simulink model "Interpolator"  (R2019a)
settings: Solver=FixedStepAuto  StartTime=0.0  StopTime=inf  FixedStep=0.001  RelTol=1e-3
settings Model: NumberOfSteps=1000  Creator=EiLit  LastModifiedBy=EiLit
settings DataIOCC: ReturnWorkspaceOutputs=off
settings DebuggingCC: ArithmeticOperatorsInVariantConditions=warning

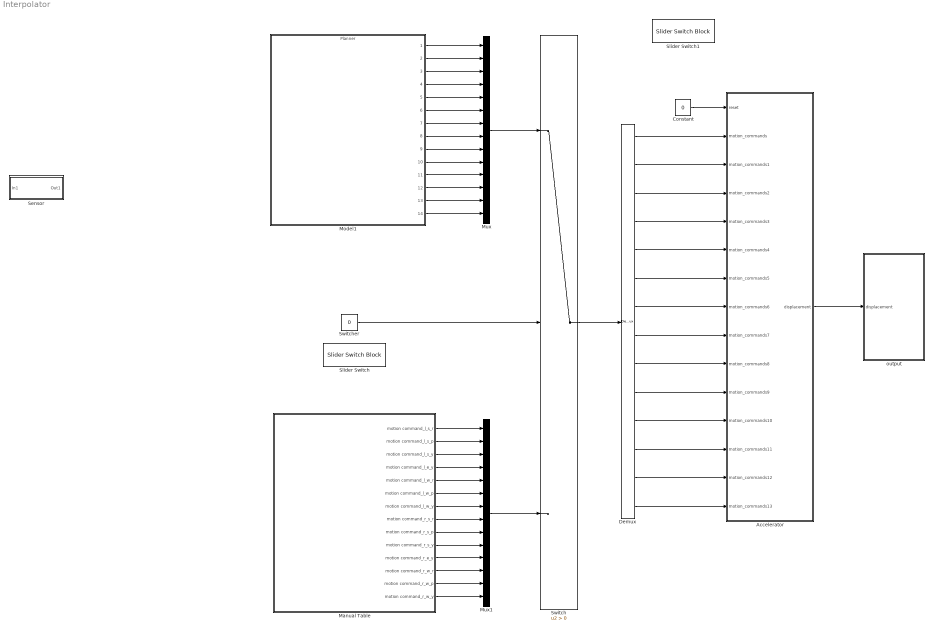
== system Interpolator ==
  Accelerator : Subsystem
  Constant : Constant  Value=0
  Demux : Demux  Outputs=14
  Manual Table : Subsystem
  Model1 : ModelReference  ModelNameDialog=Planner  SimulationMode=Normal  ModelReferenceVersion=1.6
  Mux : Mux  Inputs=14
  Mux1 : Mux  Inputs=14
  Sensor : Subsystem
  Slider Switch : SliderSwitchBlock
      settings: Values={{'Auto', 'Mannual'}, [1 0]}
  Slider Switch1 : SliderSwitchBlock
      settings: Values={{'off', 'reset'}, [0 1]}
  Switch : Switch  Criteria=u2 > Threshold
  Switcher : Constant  Value=0
  output : Subsystem
  wires:
  Accelerator/1(displacement) -> output/1(displacement)
  Switch/1 -> Demux/1
  Switcher/1 -> Switch/2
  Model1/1 -> Mux/1
  Model1/2 -> Mux/2
  Model1/3 -> Mux/3
  Model1/4 -> Mux/4
  Model1/5 -> Mux/5
  Model1/6 -> Mux/6
  Model1/7 -> Mux/7
  Model1/8 -> Mux/8
  Model1/9 -> Mux/9
  Model1/10 -> Mux/10
  Model1/11 -> Mux/11
  Model1/12 -> Mux/12
  Model1/13 -> Mux/13
  Model1/14 -> Mux/14
  Mux/1 -> Switch/1
  Mux1/1 -> Switch/3
  Manual Table/1(motion command_l_s_r) -> Mux1/1
  Manual Table/2(motion command_l_s_p) -> Mux1/2
  Manual Table/3(motion command_l_s_y) -> Mux1/3
  Manual Table/4(motion command_l_e_y) -> Mux1/4
  Manual Table/5(motion command_l_w_r) -> Mux1/5
  Manual Table/6(motion command_l_w_p) -> Mux1/6
  Manual Table/7(motion command_l_w_y) -> Mux1/7
  Manual Table/8(motion command_r_s_r) -> Mux1/8
  Manual Table/9(motion command_r_s_p) -> Mux1/9
  Manual Table/10(motion command_r_s_y) -> Mux1/10
  Manual Table/11(motion command_r_e_y) -> Mux1/11
  Manual Table/12(motion command_r_w_r) -> Mux1/12
  Manual Table/13(motion command_r_w_p) -> Mux1/13
  Manual Table/14(motion command_r_w_y) -> Mux1/14
  Demux/1 -> Accelerator/2(motion_commands)
  Demux/2 -> Accelerator/3(motion_commands1)
  Demux/3 -> Accelerator/4(motion_commands2)
  Demux/4 -> Accelerator/5(motion_commands3)
  Demux/5 -> Accelerator/6(motion_commands4)
  Demux/6 -> Accelerator/7(motion_commands5)
  Demux/7 -> Accelerator/8(motion_commands6)
  Demux/8 -> Accelerator/9(motion_commands7)
  Demux/9 -> Accelerator/10(motion_commands8)
  Demux/10 -> Accelerator/11(motion_commands9)
  Demux/11 -> Accelerator/12(motion_commands10)
  Demux/12 -> Accelerator/13(motion_commands11)
  Demux/13 -> Accelerator/14(motion_commands12)
  Demux/14 -> Accelerator/15(motion_commands13)
  Constant/1 -> Accelerator/1(reset)

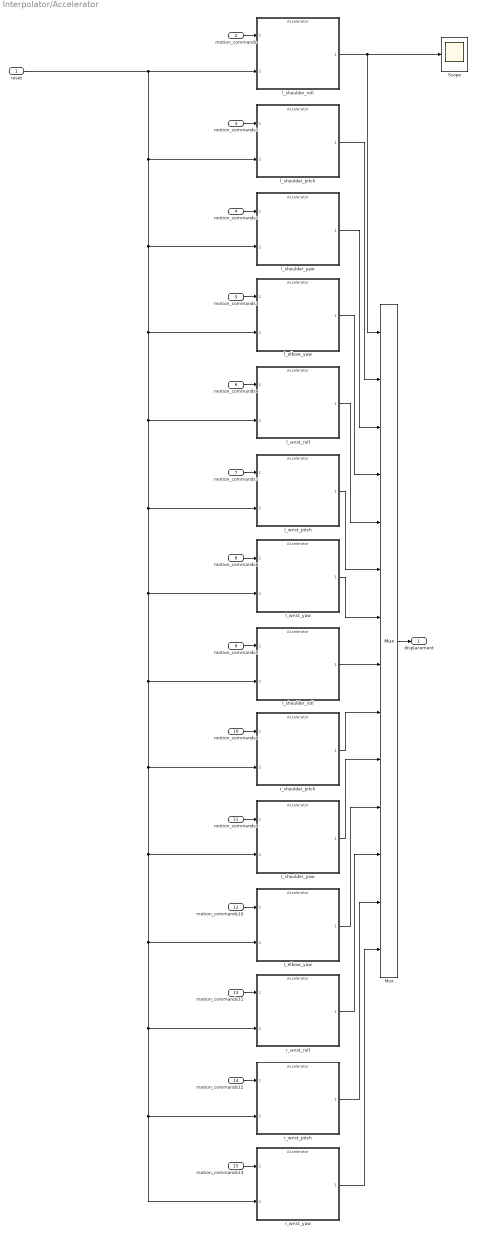
== system Interpolator/Accelerator ==
  reset : Inport
  motion_commands : Inport  Port=2
  motion_commands1 : Inport  Port=3
  motion_commands2 : Inport  Port=4
  motion_commands3 : Inport  Port=5
  motion_commands4 : Inport  Port=6
  motion_commands5 : Inport  Port=7
  motion_commands6 : Inport  Port=8
  motion_commands7 : Inport  Port=9
  motion_commands8 : Inport  Port=10
  motion_commands9 : Inport  Port=11
  motion_commands10 : Inport  Port=12
  motion_commands11 : Inport  Port=13
  motion_commands12 : Inport  Port=14
  motion_commands13 : Inport  Port=15
  Mux : Mux  Inputs=14
  Scope : Scope
  l_elbow_yaw : ModelReference  ModelNameDialog=Accelerator  SimulationMode=Normal  ModelReferenceVersion=1.104
  l_shoulder_pitch : ModelReference  ModelNameDialog=Accelerator  SimulationMode=Normal  ModelReferenceVersion=1.104
  l_shoulder_roll : ModelReference  ModelNameDialog=Accelerator  SimulationMode=Normal  ModelReferenceVersion=1.104
  l_shoulder_yaw : ModelReference  ModelNameDialog=Accelerator  SimulationMode=Normal  ModelReferenceVersion=1.104
  l_wrist_pitch : ModelReference  ModelNameDialog=Accelerator  SimulationMode=Normal  ModelReferenceVersion=1.104
  l_wrist_roll : ModelReference  ModelNameDialog=Accelerator  SimulationMode=Normal  ModelReferenceVersion=1.104
  l_wrist_yaw : ModelReference  ModelNameDialog=Accelerator  SimulationMode=Normal  ModelReferenceVersion=1.104
  r_elbow_yaw : ModelReference  ModelNameDialog=Accelerator  SimulationMode=Normal  ModelReferenceVersion=1.104
  r_shoulder_pitch : ModelReference  ModelNameDialog=Accelerator  SimulationMode=Normal  ModelReferenceVersion=1.104
  r_shoulder_roll : ModelReference  ModelNameDialog=Accelerator  SimulationMode=Normal  ModelReferenceVersion=1.104
  r_shoulder_yaw : ModelReference  ModelNameDialog=Accelerator  SimulationMode=Normal  ModelReferenceVersion=1.104
  r_wrist_pitch : ModelReference  ModelNameDialog=Accelerator  SimulationMode=Normal  ModelReferenceVersion=1.104
  r_wrist_roll : ModelReference  ModelNameDialog=Accelerator  SimulationMode=Normal  ModelReferenceVersion=1.104
  r_wrist_yaw : ModelReference  ModelNameDialog=Accelerator  SimulationMode=Normal  ModelReferenceVersion=1.104
  displacement : Outport
  wires:
  motion_commands13/1 -> r_wrist_yaw/1
  Mux/1 -> displacement/1
  l_shoulder_pitch/1 -> Mux/2
  r_shoulder_pitch/1 -> Mux/9
  r_shoulder_roll/1 -> Mux/8
  l_wrist_yaw/1 -> Mux/7
  l_wrist_pitch/1 -> Mux/6
  l_wrist_roll/1 -> Mux/5
  motion_commands/1 -> l_shoulder_roll/1
  l_elbow_yaw/1 -> Mux/4
  r_shoulder_yaw/1 -> Mux/10
  l_shoulder_yaw/1 -> Mux/3
  motion_commands7/1 -> r_shoulder_roll/1
  r_elbow_yaw/1 -> Mux/11
  r_wrist_roll/1 -> Mux/12
  r_wrist_pitch/1 -> Mux/13
  r_wrist_yaw/1 -> Mux/14
  motion_commands2/1 -> l_shoulder_yaw/1
  motion_commands12/1 -> r_wrist_pitch/1
  motion_commands11/1 -> r_wrist_roll/1
  motion_commands10/1 -> r_elbow_yaw/1
  motion_commands9/1 -> r_shoulder_yaw/1
  motion_commands1/1 -> l_shoulder_pitch/1
  motion_commands8/1 -> r_shoulder_pitch/1
  motion_commands5/1 -> l_wrist_pitch/1
  motion_commands6/1 -> l_wrist_yaw/1
  motion_commands4/1 -> l_wrist_roll/1
  motion_commands3/1 -> l_elbow_yaw/1
  reset/1 -> r_wrist_yaw/2, r_wrist_pitch/2, r_wrist_roll/2, r_elbow_yaw/2, r_shoulder_yaw/2, r_shoulder_pitch/2, r_shoulder_roll/2, l_wrist_yaw/2, l_wrist_pitch/2, l_wrist_roll/2, l_elbow_yaw/2, l_shoulder_yaw/2, l_shoulder_pitch/2, l_shoulder_roll/2
  l_shoulder_roll/1 -> Scope/1, Mux/1

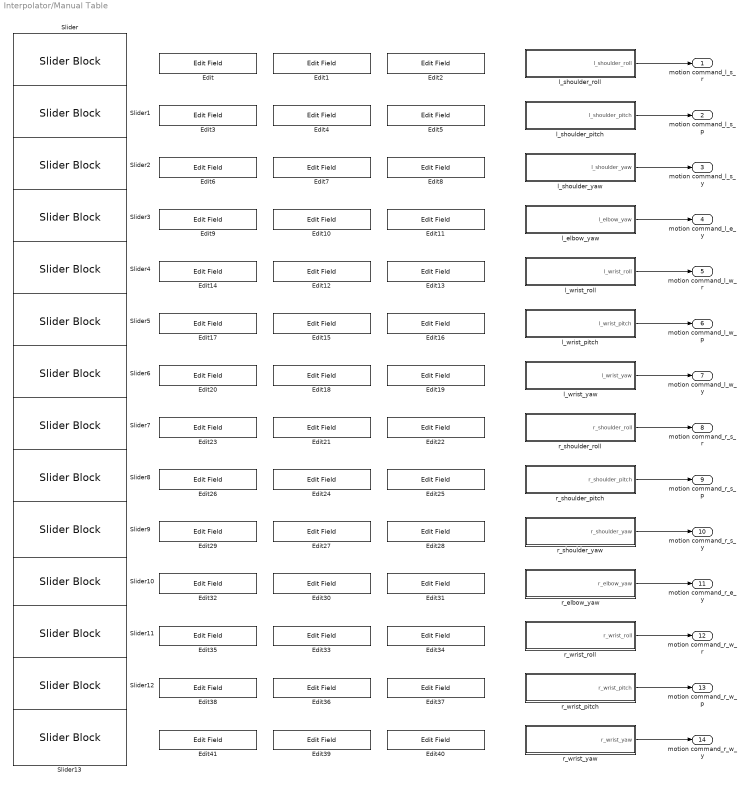
== system Interpolator/Manual Table ==
  Edit{,1..41} (42 alike) : EditField  LabelPosition=Hide  ShowInitialText=on  Alignment=Center
  Slider{,1..13} (14 alike) : SliderBlock  ScaleMin=-180  ScaleMax=180
  l_elbow_yaw : Subsystem
  l_shoulder_pitch : Subsystem
  l_shoulder_roll : Subsystem
  l_shoulder_yaw : Subsystem
  l_wrist_pitch : Subsystem
  l_wrist_roll : Subsystem
  l_wrist_yaw : Subsystem
  r_elbow_yaw : Subsystem
  r_shoulder_pitch : Subsystem
  r_shoulder_roll : Subsystem
  r_shoulder_yaw : Subsystem
  r_wrist_pitch : Subsystem
  r_wrist_roll : Subsystem
  r_wrist_yaw : Subsystem
  motion command_l_s_r : Outport
  motion command_l_s_p : Outport  Port=2
  motion command_l_s_y : Outport  Port=3
  motion command_l_e_y : Outport  Port=4
  motion command_l_w_r : Outport  Port=5
  motion command_l_w_p : Outport  Port=6
  motion command_l_w_y : Outport  Port=7
  motion command_r_s_r : Outport  Port=8
  motion command_r_s_p : Outport  Port=9
  motion command_r_s_y : Outport  Port=10
  motion command_r_e_y : Outport  Port=11
  motion command_r_w_r : Outport  Port=12
  motion command_r_w_p : Outport  Port=13
  motion command_r_w_y : Outport  Port=14
  wires:
  l_shoulder_roll/1(l_shoulder_roll) -> motion command_l_s_r/1
  l_shoulder_pitch/1(l_shoulder_pitch) -> motion command_l_s_p/1
  l_shoulder_yaw/1(l_shoulder_yaw) -> motion command_l_s_y/1
  l_elbow_yaw/1(l_elbow_yaw) -> motion command_l_e_y/1
  l_wrist_roll/1(l_wrist_roll) -> motion command_l_w_r/1
  l_wrist_pitch/1(l_wrist_pitch) -> motion command_l_w_p/1
  l_wrist_yaw/1(l_wrist_yaw) -> motion command_l_w_y/1
  r_shoulder_roll/1(r_shoulder_roll) -> motion command_r_s_r/1
  r_shoulder_pitch/1(r_shoulder_pitch) -> motion command_r_s_p/1
  r_shoulder_yaw/1(r_shoulder_yaw) -> motion command_r_s_y/1
  r_elbow_yaw/1(r_elbow_yaw) -> motion command_r_e_y/1
  r_wrist_roll/1(r_wrist_roll) -> motion command_r_w_r/1
  r_wrist_pitch/1(r_wrist_pitch) -> motion command_r_w_p/1
  r_wrist_yaw/1(r_wrist_yaw) -> motion command_r_w_y/1

== system Interpolator/Sensor ==
  In1 : Inport
  Out1 : Outport
  wires:
  In1/1 -> Out1/1

== system Interpolator/output ==
  displacement : Inport

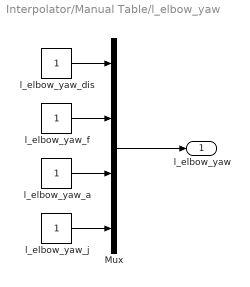
== system Interpolator/Manual Table/l_elbow_yaw ==
  Mux : Mux
  l_elbow_yaw_a : Constant
  l_elbow_yaw_dis : Constant
  l_elbow_yaw_f : Constant
  l_elbow_yaw_j : Constant
  l_elbow_yaw : Outport
  wires:
  l_elbow_yaw_dis/1 -> Mux/1
  l_elbow_yaw_f/1 -> Mux/2
  Mux/1 -> l_elbow_yaw/1
  l_elbow_yaw_a/1 -> Mux/3
  l_elbow_yaw_j/1 -> Mux/4

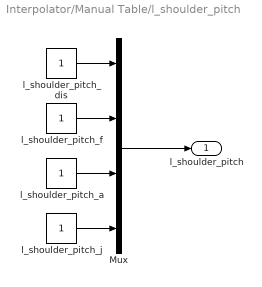
== system Interpolator/Manual Table/l_shoulder_pitch ==
  Mux : Mux
  l_shoulder_pitch_a : Constant
  l_shoulder_pitch_dis : Constant
  l_shoulder_pitch_f : Constant
  l_shoulder_pitch_j : Constant
  l_shoulder_pitch : Outport
  wires:
  l_shoulder_pitch_dis/1 -> Mux/1
  l_shoulder_pitch_f/1 -> Mux/2
  Mux/1 -> l_shoulder_pitch/1
  l_shoulder_pitch_a/1 -> Mux/3
  l_shoulder_pitch_j/1 -> Mux/4

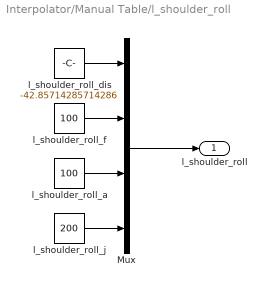
== system Interpolator/Manual Table/l_shoulder_roll ==
  Mux : Mux
  l_shoulder_roll_a : Constant  Value=100
  l_shoulder_roll_dis : Constant  Value=-42.85714285714286
  l_shoulder_roll_f : Constant  Value=100
  l_shoulder_roll_j : Constant  Value=200
  l_shoulder_roll : Outport
  wires:
  l_shoulder_roll_j/1 -> Mux/4
  l_shoulder_roll_a/1 -> Mux/3
  Mux/1 -> l_shoulder_roll/1
  l_shoulder_roll_f/1 -> Mux/2
  l_shoulder_roll_dis/1 -> Mux/1

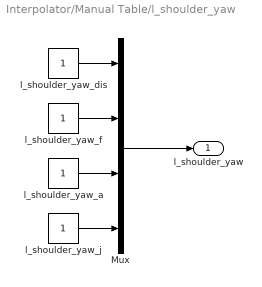
== system Interpolator/Manual Table/l_shoulder_yaw ==
  Mux : Mux
  l_shoulder_yaw_a : Constant
  l_shoulder_yaw_dis : Constant
  l_shoulder_yaw_f : Constant
  l_shoulder_yaw_j : Constant
  l_shoulder_yaw : Outport
  wires:
  l_shoulder_yaw_j/1 -> Mux/4
  l_shoulder_yaw_a/1 -> Mux/3
  Mux/1 -> l_shoulder_yaw/1
  l_shoulder_yaw_f/1 -> Mux/2
  l_shoulder_yaw_dis/1 -> Mux/1

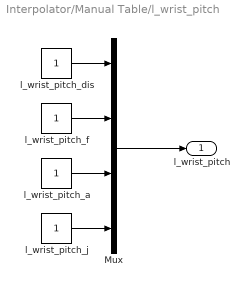
== system Interpolator/Manual Table/l_wrist_pitch ==
  Mux : Mux
  l_wrist_pitch_a : Constant
  l_wrist_pitch_dis : Constant
  l_wrist_pitch_f : Constant
  l_wrist_pitch_j : Constant
  l_wrist_pitch : Outport
  wires:
  l_wrist_pitch_dis/1 -> Mux/1
  l_wrist_pitch_f/1 -> Mux/2
  Mux/1 -> l_wrist_pitch/1
  l_wrist_pitch_a/1 -> Mux/3
  l_wrist_pitch_j/1 -> Mux/4

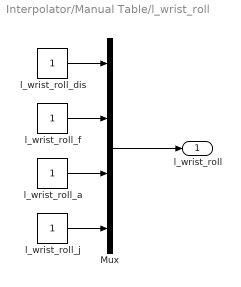
== system Interpolator/Manual Table/l_wrist_roll ==
  Mux : Mux
  l_wrist_roll_a : Constant
  l_wrist_roll_dis : Constant
  l_wrist_roll_f : Constant
  l_wrist_roll_j : Constant
  l_wrist_roll : Outport
  wires:
  l_wrist_roll_j/1 -> Mux/4
  l_wrist_roll_a/1 -> Mux/3
  Mux/1 -> l_wrist_roll/1
  l_wrist_roll_f/1 -> Mux/2
  l_wrist_roll_dis/1 -> Mux/1

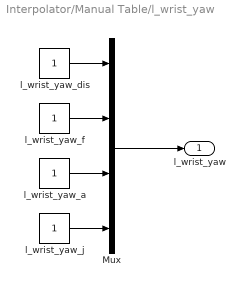
== system Interpolator/Manual Table/l_wrist_yaw ==
  Mux : Mux
  l_wrist_yaw_a : Constant
  l_wrist_yaw_dis : Constant
  l_wrist_yaw_f : Constant
  l_wrist_yaw_j : Constant
  l_wrist_yaw : Outport
  wires:
  l_wrist_yaw_j/1 -> Mux/4
  l_wrist_yaw_a/1 -> Mux/3
  Mux/1 -> l_wrist_yaw/1
  l_wrist_yaw_f/1 -> Mux/2
  l_wrist_yaw_dis/1 -> Mux/1

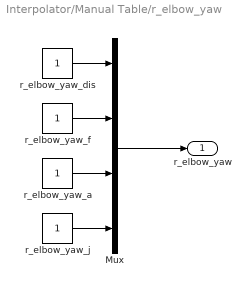
== system Interpolator/Manual Table/r_elbow_yaw ==
  Mux : Mux
  r_elbow_yaw_a : Constant
  r_elbow_yaw_dis : Constant
  r_elbow_yaw_f : Constant
  r_elbow_yaw_j : Constant
  r_elbow_yaw : Outport
  wires:
  r_elbow_yaw_j/1 -> Mux/4
  r_elbow_yaw_a/1 -> Mux/3
  Mux/1 -> r_elbow_yaw/1
  r_elbow_yaw_f/1 -> Mux/2
  r_elbow_yaw_dis/1 -> Mux/1

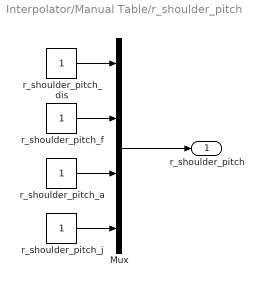
== system Interpolator/Manual Table/r_shoulder_pitch ==
  Mux : Mux
  r_shoulder_pitch_a : Constant
  r_shoulder_pitch_dis : Constant
  r_shoulder_pitch_f : Constant
  r_shoulder_pitch_j : Constant
  r_shoulder_pitch : Outport
  wires:
  r_shoulder_pitch_j/1 -> Mux/4
  r_shoulder_pitch_a/1 -> Mux/3
  Mux/1 -> r_shoulder_pitch/1
  r_shoulder_pitch_f/1 -> Mux/2
  r_shoulder_pitch_dis/1 -> Mux/1

== system Interpolator/Manual Table/r_shoulder_roll ==
  Mux : Mux
  r_shoulder_roll_a : Constant
  r_shoulder_roll_dis : Constant
  r_shoulder_roll_f : Constant
  r_shoulder_roll_j : Constant
  r_shoulder_roll : Outport
  wires:
  r_shoulder_roll_dis/1 -> Mux/1
  r_shoulder_roll_f/1 -> Mux/2
  Mux/1 -> r_shoulder_roll/1
  r_shoulder_roll_a/1 -> Mux/3
  r_shoulder_roll_j/1 -> Mux/4

== system Interpolator/Manual Table/r_shoulder_yaw ==
  Mux : Mux
  r_shoulder_yaw_a : Constant
  r_shoulder_yaw_dis : Constant
  r_shoulder_yaw_f : Constant
  r_shoulder_yaw_j : Constant
  r_shoulder_yaw : Outport
  wires:
  r_shoulder_yaw_dis/1 -> Mux/1
  r_shoulder_yaw_f/1 -> Mux/2
  Mux/1 -> r_shoulder_yaw/1
  r_shoulder_yaw_a/1 -> Mux/3
  r_shoulder_yaw_j/1 -> Mux/4

== system Interpolator/Manual Table/r_wrist_pitch ==
  Mux : Mux
  r_wrist_pitch_a : Constant
  r_wrist_pitch_dis : Constant
  r_wrist_pitch_f : Constant
  r_wrist_pitch_j : Constant
  r_wrist_pitch : Outport
  wires:
  r_wrist_pitch_j/1 -> Mux/4
  r_wrist_pitch_a/1 -> Mux/3
  Mux/1 -> r_wrist_pitch/1
  r_wrist_pitch_f/1 -> Mux/2
  r_wrist_pitch_dis/1 -> Mux/1

== system Interpolator/Manual Table/r_wrist_roll ==
  Mux : Mux
  r_wrist_roll_a : Constant
  r_wrist_roll_dis : Constant
  r_wrist_roll_f : Constant
  r_wrist_roll_j : Constant
  r_wrist_roll : Outport
  wires:
  r_wrist_roll_dis/1 -> Mux/1
  r_wrist_roll_f/1 -> Mux/2
  Mux/1 -> r_wrist_roll/1
  r_wrist_roll_a/1 -> Mux/3
  r_wrist_roll_j/1 -> Mux/4

== system Interpolator/Manual Table/r_wrist_yaw ==
  Mux : Mux
  r_wrist_yaw_a : Constant
  r_wrist_yaw_dis : Constant
  r_wrist_yaw_f : Constant
  r_wrist_yaw_j : Constant
  r_wrist_yaw : Outport
  wires:
  r_wrist_yaw_dis/1 -> Mux/1
  r_wrist_yaw_f/1 -> Mux/2
  Mux/1 -> r_wrist_yaw/1
  r_wrist_yaw_a/1 -> Mux/3
  r_wrist_yaw_j/1 -> Mux/4
